simulink model "EPLL_inverter"  (R2019b)
settings: Solver=ode45  StartTime=0.0  StopTime=0.2  MaxStep=1e-6  AbsTol=1e-6
values from neighbouring files (symbols this model uses):
  E = 400    [EPLL_inverter_params.m]
  K_vco = 1    [EPLL_inverter_params.m]
  L = 5e-3    (= 0.005)    [EPLL_inverter_params.m]
  mu_1 = 200    [EPLL_inverter_params.m]
  omega_ref = 60    [EPLL_inverter_params.m]
  omega_vco_free = 50    [EPLL_inverter_params.m]
  R = 1    [EPLL_inverter_params.m]
  tau_1 = 1/mu_2    (= 5e-05)    [EPLL_inverter_params.m]
  tau_2 = mu_3/mu_2    (= 0.02)    [EPLL_inverter_params.m]
undefined symbols (not defined in the file or in its folder): t_step
libraries: powerlib x13, powerlib_meascontrol x1
settings Model: Creator=Vogal  LastModifiedBy=mir
settings SolverCC: AutoScaleAbsTol=off  InitialStep=1e-6
settings DataIOCC: ReturnWorkspaceOutputs=off
settings OptimizationCC: LifeSpan=inf
settings DebuggingCC: AllowSymbolicDim=off  SFExecutionAtInitializationDiag=none  ArithmeticOperatorsInVariantConditions=warning
settings HardwareCC: ProdBitPerSizeT=32  ProdBitPerPtrDiffT=32  ProdWordSize=32  ProdHWDeviceType=Specified
settings SFSimCC: SimUseLocalCustomCode=off  CustomCodeUndefinedFunction=UseInterfaceOnly
settings RTWCC: RTWUseLocalCustomCode=off
settings CodeAppCC: StateflowObjectComments=on
settings SimscapeCC: SimscapeNormalizeSystem=off

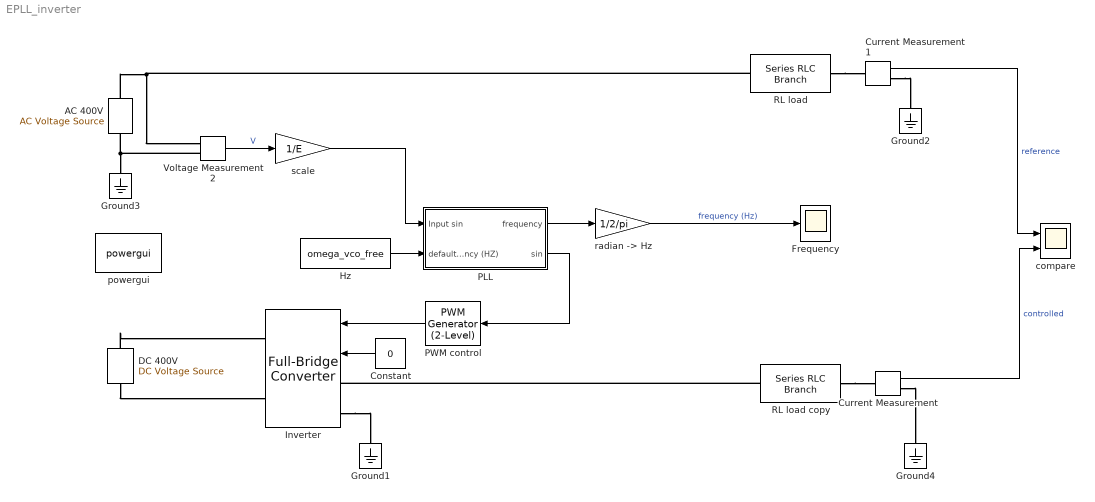
== system EPLL_inverter ==
  AC 400V : powerlib/Electrical Sources/AC Voltage Source  Amplitude=E  Phase=0  Frequency=omega_ref  SampleTime=0  Measurements=None  BusType=swing  Pref=10e3  Qref=0  Qmin=-inf  Qmax=+inf
      settings: SourceProductName=Simscape Electrical
  Constant : Constant  Value=0
  Current Measurement : powerlib/Measurements/Current Measurement  PhasorSimulation=off  OutputType=Complex  PSBequivalent=0
      settings: SourceProductName=Simscape Electrical
  Current Measurement1 : powerlib/Measurements/Current Measurement  PhasorSimulation=off  OutputType=Complex  PSBequivalent=0
      settings: SourceProductName=Simscape Electrical
  DC 400V : powerlib/Electrical Sources/DC Voltage Source  Amplitude=E  Measurements=None
      settings: SourceProductName=Simscape Electrical
  Frequency : Scope
  Ground{1..4} (4 alike) : powerlib/Elements/Ground  LConnTagsString=a
      settings: SourceProductName=Simscape Electrical
  Hz : Constant  Value=omega_vco_free
  Inverter : powerlib/Power Electronics/Full-Bridge Converter  ModelType=Switching devices  Ron=1e-3  Rs=1e6  Cs=inf  Vforward=[0,0]  Ron_Diode=1e-3  Rs_Diode=1e6  Cs_Diode=inf  Vf_Diode=1e-3  Rs_CurrentSource=inf
      settings: SourceProductName=Simscape Electrical  SourceProductBaseCode=PS
  PLL : Subsystem
  PWM control : powerlib_meascontrol/Pulse & Signal Generators/PWM Generator (2-Level)  ModulatorType=Single-phase full-bridge (4 pulses)  ModulatorMode=Unsynchronized  Fc=27*60  Pc=90  nF=27  MinMax="[ -1  1 ]"  SamplingTechnique=Natural  ModulatingSignals=off  m=0.8  Freq=60  Phase=0  Ts=0  ShowCarrierOutport=off
  RL load : powerlib/Elements/Series RLC Branch  LConnTagsString=__new0  RConnTagsString=__new0  BranchType=RL  Resistance=R  Inductance=L  SetiL0=off  InitialCurrent=0  Capacitance=1e-6  Setx0=off  InitialVoltage=0  Measurements=None
      settings: SourceProductName=Simscape Electrical
  RL load copy : powerlib/Elements/Series RLC Branch  LConnTagsString=__new0  RConnTagsString=__new0  BranchType=RL  Resistance=R  Inductance=L  SetiL0=off  InitialCurrent=0  Capacitance=1e-6  Setx0=off  InitialVoltage=0  Measurements=None
      settings: SourceProductName=Simscape Electrical
  Voltage Measurement2 : powerlib/Measurements/Voltage Measurement  PhasorSimulation=off  OutputType=Complex  PSBequivalent=0
      settings: SourceProductName=Simscape Electrical
  compare : Scope  NumInputPorts=2
  powergui : powerlib/powergui  Priority=1  SimulationMode=Discrete  SampleTime=t_step  frequency=60  Iterations=50  frequencyindice=60  Pbase=100e6  ErrMax=1e-4  UnitsV=kV  UnitsW=MW  buscounter=0  FunctionMessages=off  echomessages=off  EnableUseOfTLC=off  CurrentSourceSwitches=off  DisableSnubberDevices=off  DisableRonSwitches=off  DisableVfSwitches=off  DisplayEquations=off  AutomaticDiscreteSolvers=off  SolverType=Tustin/Backward Euler (TBE)  Interpol=off  ExternalGateDelay=off  methode=off  Ts=10  x0status=blocks  SPID=off  SwTol=0  HookPort=off  NonlinearTolerance=1e-4  nMaxIteration=100  ContinueOnMaxIteration=off  RestoreLinks=warning  ResistiveCurrentMeasurement=off  Frange=[0:2:500]  Ylog=off  Xlog=on  ShowGrid=off  save=off  variable=ZData  structure=0  ZoomFFT=off  StartTime=0.0  cycles=1  DisplayStyle=1  fundamental=60  FreqAxis=off  MaxFrequency=1000  frequencyindicesteady=1  RmsSteady=1  display=off
      settings: SourceProductName=Simscape Electrical
  "radian -> Hz" : Gain  Gain=1/2/pi
  scale : Gain  Gain=1/E
  wires:
  PLL/1(frequency) -> "radian -> Hz"/1
  "radian -> Hz"/1 -> Frequency/1  "frequency (Hz)"
  PWM control/1 -> Inverter/1
  PLL/2(sin) -> PWM control/1
  Constant/1 -> Inverter/2
  Current Measurement/1 -> compare/2  "controlled"
  Current Measurement1/1 -> compare/1  "reference"
  scale/1 -> PLL/1("Input sin ")
  Voltage Measurement2/1 -> scale/1  "V"
  Hz/1 -> PLL/2(default frequency (HZ))
  connections:
  DC 400V/RConn1 -- Inverter/RConn1
  DC 400V/LConn1 -- Inverter/RConn2
  RL load copy/LConn1 -- Inverter/LConn1
  Inverter/LConn2 -- Ground1/LConn1
  Current Measurement/RConn1 -- Ground4/LConn1
  RL load copy/RConn1 -- Current Measurement/LConn1
  Current Measurement1/RConn1 -- Ground2/LConn1
  RL load/LConn1 -- Voltage Measurement2/LConn1 -- AC 400V/RConn1
  RL load/RConn1 -- Current Measurement1/LConn1
  Voltage Measurement2/LConn2 -- Ground3/LConn1 -- AC 400V/LConn1

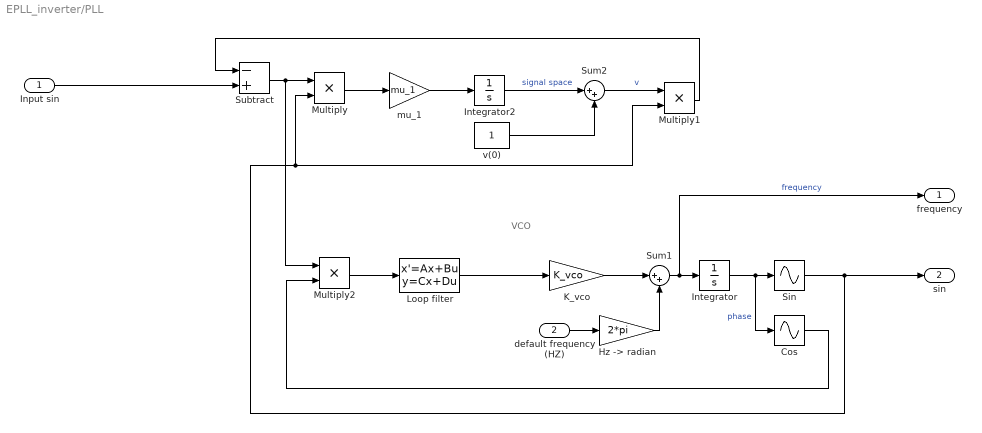
== system EPLL_inverter/PLL ==
  note: VCO
  "Input sin " : Inport
  default frequency (HZ) : Inport  Port=2
  Cos : Sin  TimeSource=Use external signal  Phase=pi/2  SampleTime=0
  "Hz -> radian" : Gain  Gain=2*pi
  Integrator : Integrator
  Integrator2 : Integrator
  K_vco : Gain  Gain=K_vco
  Loop filter : StateSpace  A=0  B=u/2/tau_1  D=tau_2*u/2/tau_1  InitialCondition=0
  Multiply : Product
  Multiply1 : Product
  Multiply2 : Product
  Sin : Sin  TimeSource=Use external signal  SampleTime=0
  Subtract : Sum  Inputs=-+
  Sum1 : Sum  Inputs=|++
  Sum2 : Sum  Inputs=|++
  mu_1 : Gain  Gain=mu_1
  v(0) : Constant
  frequency : Outport
  sin : Outport  Port=2
  wires:
  "Input sin "/1 -> Subtract/2
  Multiply1/1 -> Subtract/1
  K_vco/1 -> Sum1/1
  "Hz -> radian"/1 -> Sum1/2
  Cos/1 -> Multiply2/2
  Integrator/1 -> Cos/1, Sin/1  "phase"
  Subtract/1 -> Multiply2/1, Multiply/1
  Sum1/1 -> frequency/1, Integrator/1  "frequency"
  Loop filter/1 -> K_vco/1
  mu_1/1 -> Integrator2/1
  Sin/1 -> sin/1, Multiply/2, Multiply1/2
  Multiply/1 -> mu_1/1
  Multiply2/1 -> Loop filter/1
  Integrator2/1 -> Sum2/1  "signal space"
  Sum2/1 -> Multiply1/1  "v"
  v(0)/1 -> Sum2/2
  default frequency (HZ)/1 -> "Hz -> radian"/1
